simulink model "control_pmsm_multiple"  (R2023a)
settings: Solver=FixedStepAuto  StartTime=0.0  StopTime=0.3  RelTol=1e-3  EnableMultiTasking=on
undefined symbols (not defined in the file): ControlModes, EstimationVelocityModes
settings Model: DataDictionary=EmbeddedBoardDD.sldd  SimulationMode=accelerator  Creator=upattacini  LastModifiedBy=mfussi
settings SolverCC: AllowMultiTaskInputOutput=on  AutoInsertRateTranBlk=on  InsertRTBMode=Never (minimum delay)  EnableFixedStepZeroCrossing=on
settings DataIOCC: SaveOutput=off  DSMLogging=off  SaveTime=off  ReturnWorkspaceOutputs=off
settings OptimizationCC: SimCompilerOptimization=on
settings DebuggingCC: ParameterPrecisionLossMsg=none  UnconnectedInputMsg=warning  UnconnectedOutputMsg=warning  UnconnectedLineMsg=warning
settings ModelReferenceCC: EnableRefExpFcnMdlSchedulingChecks=on
settings RTWCC: DLArmComputeVersion=19.05

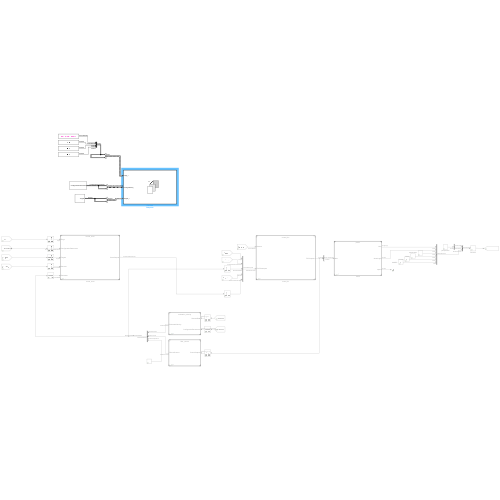
[thumbnail: Simulink's stored preview of the top-level diagram]
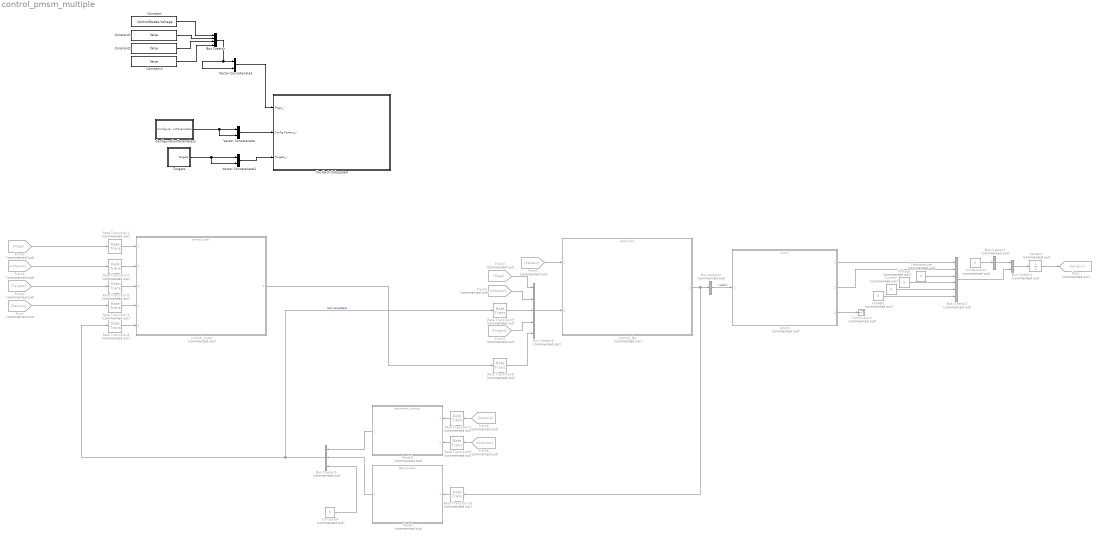
== system control_pmsm_multiple ==
  Bus Creator : BusCreator  Inputs=4  OutDataTypeStr=Bus: Flags  NonVirtualBus=on
      settings: InheritFromInputs=off
  Bus Creator1 : BusCreator  Commented=on  Inputs=2  OutDataTypeStr=Bus: SensorsData  NonVirtualBus=on
      settings: InheritFromInputs=off
  Bus Creator2 : BusCreator  Commented=on  Inputs=6  OutDataTypeStr=Bus: MotorSensors  NonVirtualBus=on
      settings: InheritFromInputs=off
  Bus Creator3 : BusCreator  Commented=on  Inputs=1  OutDataTypeStr=Bus: JointPositions  NonVirtualBus=on
      settings: InheritFromInputs=off
  Bus Creator5 : BusCreator  Commented=on  Inputs=3  OutDataTypeStr=Bus: EstimatedData  NonVirtualBus=on
      settings: InheritFromInputs=off
  Bus Creator6 : BusCreator  Commented=on  Inputs=5  OutDataTypeStr=Bus: FOCSlowInputs  NonVirtualBus=on
      settings: InheritFromInputs=off
  Bus Selector : BusSelector  Commented=on  OutputSignals=Vabc
  ConfigurationParameters : Subsystem
  Constant : Constant  Value=ControlModes.Voltage  OutDataTypeStr=Enum: ControlModes  LockScale=on
  Constant1 : Constant  Value=false  OutDataTypeStr=boolean  LockScale=on
  Constant2 : Constant  Value=false  OutDataTypeStr=boolean  LockScale=on
  Constant3 : Constant  Value=false  OutDataTypeStr=boolean  LockScale=on
  Constant4 : Constant  Commented=on  Value=0  OutDataTypeStr=Bus: MotorTemperature
  Current : Constant  Commented=on  Value=0  OutDataTypeStr=single
  For Each Subsystem : Subsystem  TreatAsAtomicUnit=on
  From : From  Commented=on  GotoTag=Sensors
  From1 : From  Commented=on  GotoTag=Sensors
  From2 : From  Commented=on  GotoTag=Targets
  From3 : From  Commented=on  GotoTag=Targets
  From4 : From  Commented=on  GotoTag=Configuration
  From5 : From  Commented=on  GotoTag=Configuration
  From6 : From  Commented=on  GotoTag=Flags
  From7 : From  Commented=on  GotoTag=Flags
  From8 : From  Commented=on  GotoTag=Configuration
  From9 : From  Commented=on  GotoTag=Sensors
  Goto : Goto  Commented=on  GotoTag=Sensors
  Model : ModelReference  Commented=on  ModelNameDialog=filter_current.slx  SimulationMode=Normal  ModelReferenceVersion=5.1
  Model1 : ModelReference  Commented=on  ModelNameDialog=estimation_velocity.slx  SimulationMode=Normal  ModelReferenceVersion=5.1
  Rate Transition{1..10} (10 alike) : RateTransition  Commented=on  Deterministic=off
  Sensors : UnitDelay  Commented=on  SampleTime=-1  HasFrameUpgradeWarning=on
  Targets : Subsystem
  Temperature : Constant  Commented=on  Value=0  OutDataTypeStr=single
  Terminator1 : Terminator  Commented=on
  Vector Concatenate : Concatenate
  Vector Concatenate1 : Concatenate
  Vector Concatenate2 : Concatenate
  Voltage : Constant  Commented=on  Value=0  OutDataTypeStr=single
  control_foc : ModelReference  Commented=on  ModelNameDialog=control_foc.slx  SimulationMode=Normal  ModelReferenceVersion=5.12
  control_outer : ModelReference  Commented=on  ModelNameDialog=control_outer.slx  SimulationMode=Normal  ModelReferenceVersion=5.5
  hallABC : Constant  Commented=on  Value=0  OutDataTypeStr=uint8
  jointposition : Constant  Commented=on  Value=0  OutDataTypeStr=single
  pmsm : ModelReference  Commented=on  ModelNameDialog=pmsm.slx  SimulationMode=Normal  ModelReferenceVersion=6.0
  wires:
  control_foc/1 -> Rate Transition10/1, Bus Selector/1
  Bus Selector/1 -> pmsm/1  "<Vabc>"
  Constant/1 -> Bus Creator/1
  Bus Creator3/1 -> Bus Creator1/1
  jointposition/1 -> Bus Creator3/1
  pmsm/1 -> Bus Creator2/1
  Temperature/1 -> Bus Creator2/3
  Voltage/1 -> Bus Creator2/4
  Current/1 -> Bus Creator2/5
  hallABC/1 -> Bus Creator2/6
  pmsm/3 -> Terminator1/1
  Bus Creator2/1 -> Bus Creator1/2
  Bus Creator1/1 -> Sensors/1
  ConfigurationParameters/1(ConfigurationParameters) -> Vector Concatenate/2, Vector Concatenate/1
  pmsm/2 -> Bus Creator2/2
  Sensors/1 -> Goto/1
  From6/1 -> Rate Transition1/1
  Rate Transition1/1 -> control_outer/1
  Rate Transition2/1 -> control_outer/2
  From4/1 -> Rate Transition2/1
  Rate Transition3/1 -> control_outer/4
  From/1 -> Rate Transition3/1
  Rate Transition4/1 -> control_outer/5
  Rate Transition5/1 -> control_outer/3
  From2/1 -> Rate Transition5/1
  control_outer/1 -> Rate Transition6/1
  Bus Creator6/1 -> control_foc/2
  From3/1 -> Bus Creator6/4
  Rate Transition6/1 -> Bus Creator6/5
  Bus Creator5/1 -> Rate Transition9/1, Rate Transition4/1  "EstimatedData"
  From5/1 -> Bus Creator6/2
  From7/1 -> Bus Creator6/1
  From1/1 -> control_foc/1
  Constant1/1 -> Bus Creator/2
  Constant2/1 -> Bus Creator/3
  Model1/1 -> Bus Creator5/1
  Model/1 -> Bus Creator5/2
  From8/1 -> Rate Transition8/1
  From9/1 -> Rate Transition7/1
  Rate Transition7/1 -> Model1/1
  Rate Transition8/1 -> Model1/2
  Rate Transition9/1 -> Bus Creator6/3
  Rate Transition10/1 -> Model/1
  Constant3/1 -> Bus Creator/4
  Constant4/1 -> Bus Creator5/3
  Vector Concatenate/1 -> For Each Subsystem/2(Config Params_i)
  Bus Creator/1 -> Vector Concatenate1/2, Vector Concatenate1/1
  Vector Concatenate1/1 -> For Each Subsystem/1(Flags_i)
  Vector Concatenate2/1 -> For Each Subsystem/3(Targets_i)
  Targets/1(Targets) -> Vector Concatenate2/2, Vector Concatenate2/1

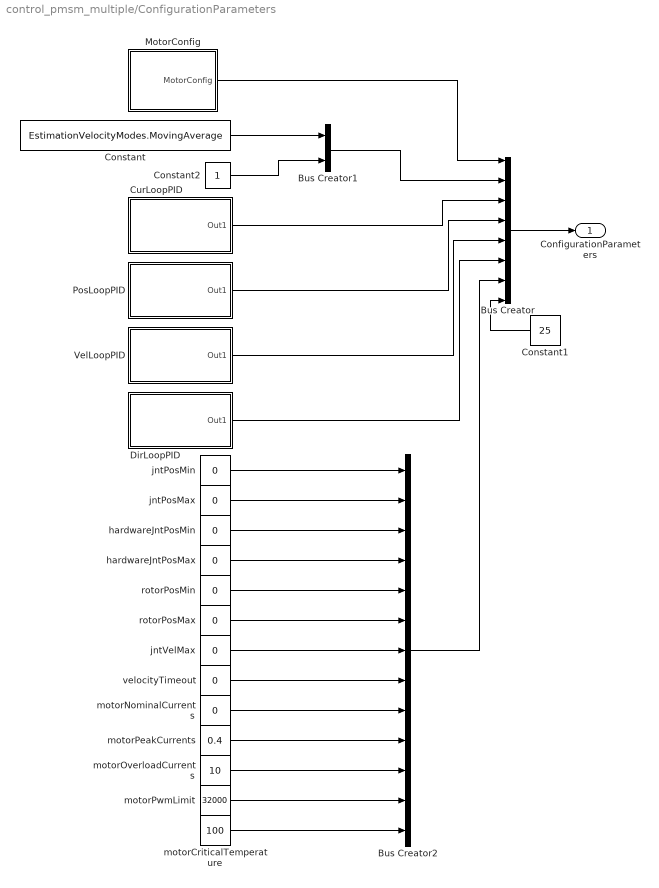
== system control_pmsm_multiple/ConfigurationParameters ==
  Bus Creator : BusCreator  Inputs=8  OutDataTypeStr=Bus: ConfigurationParameters  NonVirtualBus=on
      settings: InheritFromInputs=off
  Bus Creator1 : BusCreator  Inputs=2  OutDataTypeStr=Bus: EstimationConfig  NonVirtualBus=on
      settings: InheritFromInputs=off
  Bus Creator2 : BusCreator  Inputs=13  OutDataTypeStr=Bus: Thresholds  NonVirtualBus=on
      settings: InheritFromInputs=off
  Constant : Constant  Value=EstimationVelocityModes.MovingAverage  OutDataTypeStr=Enum: EstimationVelocityModes
  Constant1 : Constant  Value=25  OutDataTypeStr=single
  Constant2 : Constant  OutDataTypeStr=single
  CurLoopPID : Subsystem  mask{OutMax=0, OutMin=0, P=2, I=500, D=0, N=10, I0=0, D0=0, shift_factor=0}
      mask prompts: shift_factor "Shift Factor"
  DirLoopPID : Subsystem  mask{OutMax=0, OutMin=0, P=0, I=0, D=0, N=0, I0=0, D0=0, shift_factor=0}
      mask prompts: shift_factor "Shift Factor"
  MotorConfig : Subsystem  mask{has_hall_sens=true, has_quadrature_encoder=true, has_speed_quadrature_encoder=false, has_torque_sens=false, use_index=true, enable_verbosity=false, rotor_encoder_resolution=16000, rotor_index_offset=0, encoder_tolerance=0, pole_pairs=7, reduction=1, Kbemf=0, Rphase=0, Imin=-10, Imax=10, Vcc=24, Vmax=24, R=29.5, L=200, Rt=50, tau=200}
      mask prompts: R "Motor Resistance"; L "Motor Inductance"; Rt "Thermal Resistance"; tau "Thermal Time Constant"
  PosLoopPID : Subsystem  mask{OutMax=0, OutMin=0, P=0, I=0, D=0, N=0, I0=0, D0=0, shift_factor=0}
      mask prompts: shift_factor "Shift Factor"
  VelLoopPID : Subsystem  mask{OutMax=0, OutMin=0, P=0, I=0, D=0, N=0, I0=0, D0=0, shift_factor=0}
      mask prompts: shift_factor "Shift Factor"
  hardwareJntPosMax : Constant  Value=0  OutDataTypeStr=single
  hardwareJntPosMin : Constant  Value=0  OutDataTypeStr=single
  jntPosMax : Constant  Value=0  OutDataTypeStr=single
  jntPosMin : Constant  Value=0  OutDataTypeStr=single
  jntVelMax : Constant  Value=0  OutDataTypeStr=single
  motorCriticalTemperature : Constant  Value=100  OutDataTypeStr=single
  motorNominalCurrents : Constant  Value=0  OutDataTypeStr=single
  motorOverloadCurrents : Constant  Value=10  OutDataTypeStr=single
  motorPeakCurrents : Constant  Value=0.4  OutDataTypeStr=single
  motorPwmLimit : Constant  Value=32000  OutDataTypeStr=uint32
  rotorPosMax : Constant  Value=0  OutDataTypeStr=single
  rotorPosMin : Constant  Value=0  OutDataTypeStr=single
  velocityTimeout : Constant  Value=0  OutDataTypeStr=uint32
  ConfigurationParameters : Outport
  wires:
  Bus Creator/1 -> ConfigurationParameters/1
  Constant/1 -> Bus Creator1/1
  jntPosMin/1 -> Bus Creator2/1
  jntPosMax/1 -> Bus Creator2/2
  hardwareJntPosMin/1 -> Bus Creator2/3
  hardwareJntPosMax/1 -> Bus Creator2/4
  rotorPosMin/1 -> Bus Creator2/5
  rotorPosMax/1 -> Bus Creator2/6
  jntVelMax/1 -> Bus Creator2/7
  velocityTimeout/1 -> Bus Creator2/8
  motorNominalCurrents/1 -> Bus Creator2/9
  motorPeakCurrents/1 -> Bus Creator2/10
  motorOverloadCurrents/1 -> Bus Creator2/11
  motorPwmLimit/1 -> Bus Creator2/12
  Bus Creator1/1 -> Bus Creator/2
  PosLoopPID/1(Out1) -> Bus Creator/4
  CurLoopPID/1(Out1) -> Bus Creator/3
  VelLoopPID/1(Out1) -> Bus Creator/5
  MotorConfig/1(MotorConfig) -> Bus Creator/1
  DirLoopPID/1(Out1) -> Bus Creator/6
  Bus Creator2/1 -> Bus Creator/7
  Constant1/1 -> Bus Creator/8
  motorCriticalTemperature/1 -> Bus Creator2/13
  Constant2/1 -> Bus Creator1/2

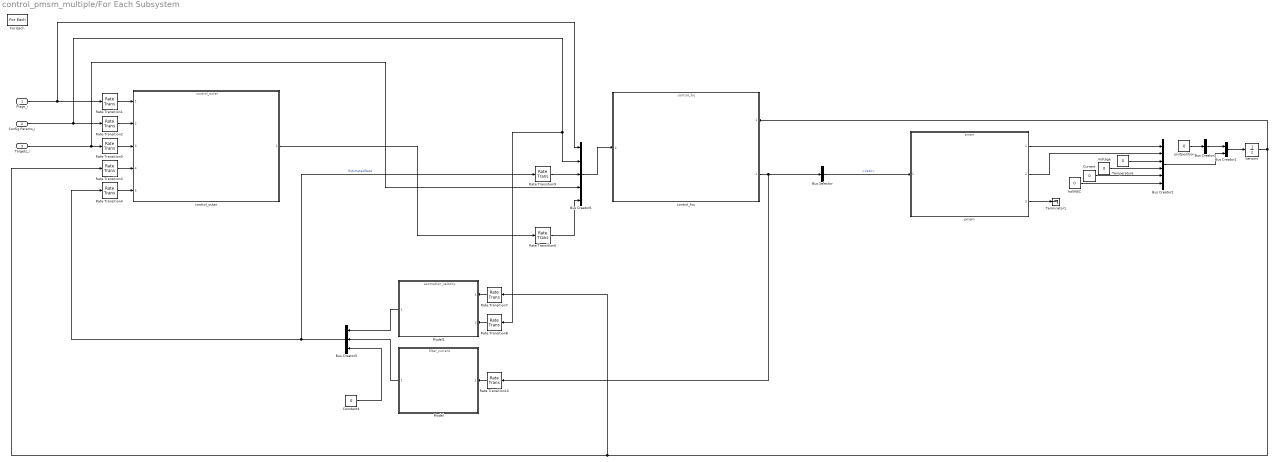
== system control_pmsm_multiple/For Each Subsystem ==
  Flags_i : Inport  OutDataTypeStr=Bus: Flags  Partition=on  PartitionDimension=1  PartitionWidth=1  PartitionOffset=0
  Config Params_i : Inport  Port=2  Partition=on  PartitionDimension=1  PartitionWidth=1  PartitionOffset=0
  Targets_i : Inport  Port=3  Partition=on  PartitionDimension=1  PartitionWidth=1  PartitionOffset=0
  Bus Creator1 : BusCreator  Inputs=2  OutDataTypeStr=Bus: SensorsData  NonVirtualBus=on
      settings: InheritFromInputs=off
  Bus Creator2 : BusCreator  Inputs=6  OutDataTypeStr=Bus: MotorSensors  NonVirtualBus=on
      settings: InheritFromInputs=off
  Bus Creator3 : BusCreator  Inputs=1  OutDataTypeStr=Bus: JointPositions  NonVirtualBus=on
      settings: InheritFromInputs=off
  Bus Creator5 : BusCreator  Inputs=3  OutDataTypeStr=Bus: EstimatedData  NonVirtualBus=on
      settings: InheritFromInputs=off
  Bus Creator6 : BusCreator  Inputs=5  OutDataTypeStr=Bus: FOCSlowInputs  NonVirtualBus=on
      settings: InheritFromInputs=off
  Bus Selector : BusSelector  OutputSignals=Vabc
  Constant4 : Constant  Value=0  OutDataTypeStr=Bus: MotorTemperature
  Current : Constant  Value=0  OutDataTypeStr=single
  For Each : ForEach  DisableCoverage=on
  Model : ModelReference  ModelNameDialog=filter_current.slx  ModelReferenceVersion=5.1
  Model1 : ModelReference  ModelNameDialog=estimation_velocity.slx  ModelReferenceVersion=5.1
  Rate Transition{1..10} (10 alike) : RateTransition  Deterministic=off
  Sensors : UnitDelay  SampleTime=-1  HasFrameUpgradeWarning=on
  Temperature : Constant  Value=0  OutDataTypeStr=single
  Terminator1 : Terminator
  Voltage : Constant  Value=0  OutDataTypeStr=single
  control_foc : ModelReference  ModelNameDialog=control_foc.slx  ModelReferenceVersion=5.12
      settings: PortSchema="{\"entries\":[{\"content\":{\"sides\":[{\"content\":{\"connectorIds\":[\"In2\"]},\"type\":\"ConnectorPlacement.EquallySpacedRectSide\",\"uuid\":\"ad3e0007-7e1a-45e3-9c4b-8557c15e59c9\"},{\"content\":{\"connectorIds\":[\"In1\",\"Out1\"],\"side\":\"RIGHT\"},\"type\":\"ConnectorPlacement.EquallySpacedRectSide\",\"uuid\":\"9939f2ed-714d-478a-b916-4c98246d3dad\"},{\"content\":{\"side\":\"TOP\"},\"type\":\"ConnectorPlacement.EquallySpacedRectSide\",\"uuid\":\"1f2bf02e-7550-4331-be09-78a4da3cd08c\"}]},\"type\":\"ConnectorPlacement.EquallySpacedConnector\",\"uuid\":\"c84d0359-7250-4a6f-b291-6b1b96be2690\"}],\"packageUris\":[\"http://schema.mathworks.com/mf0/Connector/R2020b\"],\"version\":\"1.0\"}"
  control_outer : ModelReference  ModelNameDialog=control_outer.slx  ModelReferenceVersion=5.5
  hallABC : Constant  Value=0  OutDataTypeStr=uint8
  jointposition : Constant  Value=0  OutDataTypeStr=single
  pmsm : ModelReference  ModelNameDialog=pmsm.slx  ModelReferenceVersion=6.0
  wires:
  Rate Transition8/1 -> Model1/2
  Flags_i/1 -> Rate Transition1/1, Bus Creator6/1
  Constant4/1 -> Bus Creator5/3
  Rate Transition9/1 -> Bus Creator6/3
  Bus Creator6/1 -> control_foc/2
  Rate Transition2/1 -> control_outer/2
  Sensors/1 -> Rate Transition7/1, Rate Transition3/1, control_foc/1
  Config Params_i/1 -> Rate Transition2/1, Bus Creator6/2, Rate Transition8/1
  Targets_i/1 -> Bus Creator6/4, Rate Transition5/1
  Rate Transition4/1 -> control_outer/5
  Model/1 -> Bus Creator5/2
  control_outer/1 -> Rate Transition6/1
  Rate Transition6/1 -> Bus Creator6/5
  Rate Transition7/1 -> Model1/1
  Bus Creator5/1 -> Rate Transition9/1, Rate Transition4/1  "EstimatedData"
  Rate Transition5/1 -> control_outer/3
  Rate Transition1/1 -> control_outer/1
  Rate Transition10/1 -> Model/1
  Rate Transition3/1 -> control_outer/4
  Model1/1 -> Bus Creator5/1
  control_foc/1 -> Bus Selector/1, Rate Transition10/1
  Bus Selector/1 -> pmsm/1  "<Vabc>"
  pmsm/2 -> Bus Creator2/2
  Bus Creator2/1 -> Bus Creator1/2
  Current/1 -> Bus Creator2/5
  Temperature/1 -> Bus Creator2/3
  Voltage/1 -> Bus Creator2/4
  pmsm/1 -> Bus Creator2/1
  jointposition/1 -> Bus Creator3/1
  Bus Creator3/1 -> Bus Creator1/1
  pmsm/3 -> Terminator1/1
  Bus Creator1/1 -> Sensors/1
  hallABC/1 -> Bus Creator2/6

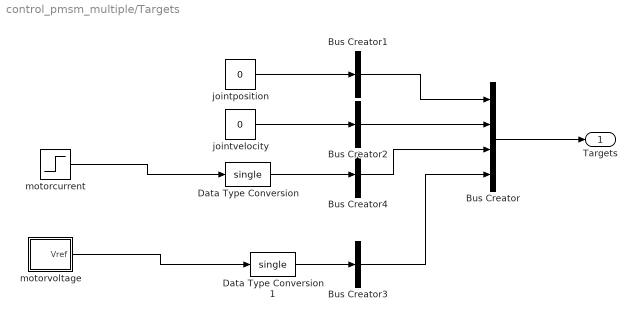
== system control_pmsm_multiple/Targets ==
  Bus Creator : BusCreator  Inputs=4  OutDataTypeStr=Bus: Targets  NonVirtualBus=on
      settings: InheritFromInputs=off
  Bus Creator1 : BusCreator  Inputs=1  OutDataTypeStr=Bus: JointPositions  NonVirtualBus=on
      settings: InheritFromInputs=off
  Bus Creator2 : BusCreator  Inputs=1  OutDataTypeStr=Bus: JointVelocities  NonVirtualBus=on
      settings: InheritFromInputs=off
  Bus Creator3 : BusCreator  Inputs=1  OutDataTypeStr=Bus: MotorVoltage  NonVirtualBus=on
      settings: InheritFromInputs=off
  Bus Creator4 : BusCreator  Inputs=1  OutDataTypeStr=Bus: MotorCurrent  NonVirtualBus=on
      settings: InheritFromInputs=off
  Data Type Conversion : DataTypeConversion  OutDataTypeStr=single  SaturateOnIntegerOverflow=off  RndMeth=Floor
  Data Type Conversion1 : DataTypeConversion  OutDataTypeStr=single  SaturateOnIntegerOverflow=off  RndMeth=Floor
  jointposition : Constant  Value=0  OutDataTypeStr=single
  jointvelocity : Constant  Value=0  OutDataTypeStr=single
  motorcurrent : Step  Time=0.1  After=0.8  SampleTime=0
  motorvoltage : Subsystem
  Targets : Outport
  wires:
  Bus Creator/1 -> Targets/1
  jointposition/1 -> Bus Creator1/1
  Bus Creator1/1 -> Bus Creator/1
  Bus Creator2/1 -> Bus Creator/2
  Bus Creator3/1 -> Bus Creator/4
  Bus Creator4/1 -> Bus Creator/3
  jointvelocity/1 -> Bus Creator2/1
  Data Type Conversion1/1 -> Bus Creator3/1
  Data Type Conversion/1 -> Bus Creator4/1
  motorcurrent/1 -> Data Type Conversion/1
  motorvoltage/1(Vref) -> Data Type Conversion1/1

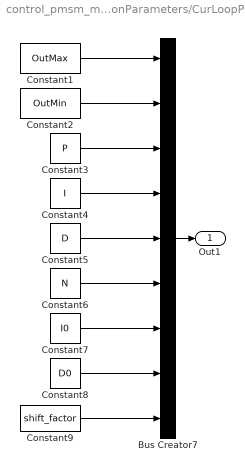
== system control_pmsm_multiple/ConfigurationParameters/CurLoopPID ==
  Bus Creator7 : BusCreator  Inputs=9  OutDataTypeStr=Bus: PIDConfig  NonVirtualBus=on
      settings: InheritFromInputs=off
  Constant1 : Constant  Value=OutMax  OutDataTypeStr=single
  Constant2 : Constant  Value=OutMin  OutDataTypeStr=single
  Constant3 : Constant  Value=P  OutDataTypeStr=single
  Constant4 : Constant  Value=I  OutDataTypeStr=single
  Constant5 : Constant  Value=D  OutDataTypeStr=single
  Constant6 : Constant  Value=N  OutDataTypeStr=single
  Constant7 : Constant  Value=I0  OutDataTypeStr=single
  Constant8 : Constant  Value=D0  OutDataTypeStr=single
  Constant9 : Constant  Value=shift_factor  OutDataTypeStr=uint8
  Out1 : Outport
  wires:
  Constant9/1 -> Bus Creator7/9
  Constant5/1 -> Bus Creator7/5
  Bus Creator7/1 -> Out1/1
  Constant8/1 -> Bus Creator7/8
  Constant2/1 -> Bus Creator7/2
  Constant4/1 -> Bus Creator7/4
  Constant7/1 -> Bus Creator7/7
  Constant1/1 -> Bus Creator7/1
  Constant3/1 -> Bus Creator7/3
  Constant6/1 -> Bus Creator7/6

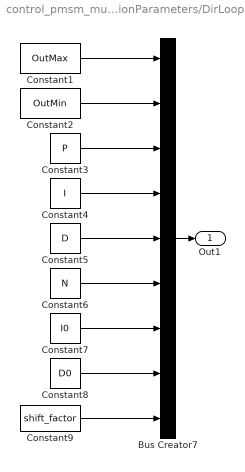
== system control_pmsm_multiple/ConfigurationParameters/DirLoopPID ==
  Bus Creator7 : BusCreator  Inputs=9  OutDataTypeStr=Bus: PIDConfig  NonVirtualBus=on
      settings: InheritFromInputs=off
  Constant1 : Constant  Value=OutMax  OutDataTypeStr=single
  Constant2 : Constant  Value=OutMin  OutDataTypeStr=single
  Constant3 : Constant  Value=P  OutDataTypeStr=single
  Constant4 : Constant  Value=I  OutDataTypeStr=single
  Constant5 : Constant  Value=D  OutDataTypeStr=single
  Constant6 : Constant  Value=N  OutDataTypeStr=single
  Constant7 : Constant  Value=I0  OutDataTypeStr=single
  Constant8 : Constant  Value=D0  OutDataTypeStr=single
  Constant9 : Constant  Value=shift_factor  OutDataTypeStr=uint8
  Out1 : Outport
  wires:
  Constant6/1 -> Bus Creator7/6
  Constant3/1 -> Bus Creator7/3
  Constant1/1 -> Bus Creator7/1
  Constant7/1 -> Bus Creator7/7
  Constant4/1 -> Bus Creator7/4
  Constant2/1 -> Bus Creator7/2
  Constant8/1 -> Bus Creator7/8
  Bus Creator7/1 -> Out1/1
  Constant5/1 -> Bus Creator7/5
  Constant9/1 -> Bus Creator7/9

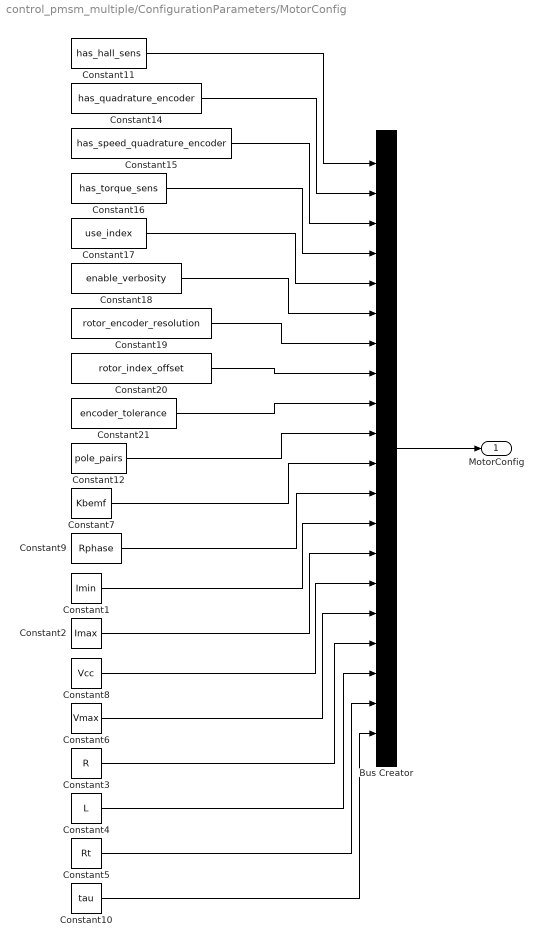
== system control_pmsm_multiple/ConfigurationParameters/MotorConfig ==
  Bus Creator : BusCreator  Inputs=20  OutDataTypeStr=Bus: MotorConfig  NonVirtualBus=on
      settings: InheritFromInputs=off
  Constant1 : Constant  Value=Imin  OutDataTypeStr=single
  Constant10 : Constant  Value=tau  OutDataTypeStr=single
  Constant11 : Constant  Value=has_hall_sens  OutDataTypeStr=boolean
  Constant12 : Constant  Value=pole_pairs  OutDataTypeStr=uint8
  Constant14 : Constant  Value=has_quadrature_encoder  OutDataTypeStr=boolean
  Constant15 : Constant  Value=has_speed_quadrature_encoder  OutDataTypeStr=boolean
  Constant16 : Constant  Value=has_torque_sens  OutDataTypeStr=boolean
  Constant17 : Constant  Value=use_index  OutDataTypeStr=boolean
  Constant18 : Constant  Value=enable_verbosity  OutDataTypeStr=boolean
  Constant19 : Constant  Value=rotor_encoder_resolution  OutDataTypeStr=int16
  Constant2 : Constant  Value=Imax  OutDataTypeStr=single
  Constant20 : Constant  Value=rotor_index_offset  OutDataTypeStr=int16
  Constant21 : Constant  Value=encoder_tolerance  OutDataTypeStr=uint8
  Constant3 : Constant  Value=R  OutDataTypeStr=single
  Constant4 : Constant  Value=L  OutDataTypeStr=single
  Constant5 : Constant  Value=Rt  OutDataTypeStr=single
  Constant6 : Constant  Value=Vmax  OutDataTypeStr=single
  Constant7 : Constant  Value=Kbemf  OutDataTypeStr=single
  Constant8 : Constant  Value=Vcc  OutDataTypeStr=single
  Constant9 : Constant  Value=Rphase  OutDataTypeStr=single
  MotorConfig : Outport
  wires:
  Bus Creator/1 -> MotorConfig/1
  Constant20/1 -> Bus Creator/8
  Constant19/1 -> Bus Creator/7
  Constant21/1 -> Bus Creator/9
  Constant15/1 -> Bus Creator/3
  Constant18/1 -> Bus Creator/6
  Constant14/1 -> Bus Creator/2
  Constant16/1 -> Bus Creator/4
  Constant17/1 -> Bus Creator/5
  Constant12/1 -> Bus Creator/10
  Constant11/1 -> Bus Creator/1
  Constant7/1 -> Bus Creator/11
  Constant9/1 -> Bus Creator/12
  Constant1/1 -> Bus Creator/13
  Constant2/1 -> Bus Creator/14
  Constant8/1 -> Bus Creator/15
  Constant6/1 -> Bus Creator/16
  Constant3/1 -> Bus Creator/17
  Constant4/1 -> Bus Creator/18
  Constant5/1 -> Bus Creator/19
  Constant10/1 -> Bus Creator/20

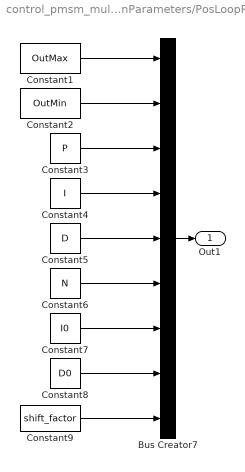
== system control_pmsm_multiple/ConfigurationParameters/PosLoopPID ==
  Bus Creator7 : BusCreator  Inputs=9  OutDataTypeStr=Bus: PIDConfig  NonVirtualBus=on
      settings: InheritFromInputs=off
  Constant1 : Constant  Value=OutMax  OutDataTypeStr=single
  Constant2 : Constant  Value=OutMin  OutDataTypeStr=single
  Constant3 : Constant  Value=P  OutDataTypeStr=single
  Constant4 : Constant  Value=I  OutDataTypeStr=single
  Constant5 : Constant  Value=D  OutDataTypeStr=single
  Constant6 : Constant  Value=N  OutDataTypeStr=single
  Constant7 : Constant  Value=I0  OutDataTypeStr=single
  Constant8 : Constant  Value=D0  OutDataTypeStr=single
  Constant9 : Constant  Value=shift_factor  OutDataTypeStr=uint8
  Out1 : Outport
  wires:
  Constant6/1 -> Bus Creator7/6
  Constant3/1 -> Bus Creator7/3
  Constant1/1 -> Bus Creator7/1
  Constant7/1 -> Bus Creator7/7
  Constant4/1 -> Bus Creator7/4
  Constant2/1 -> Bus Creator7/2
  Constant8/1 -> Bus Creator7/8
  Bus Creator7/1 -> Out1/1
  Constant5/1 -> Bus Creator7/5
  Constant9/1 -> Bus Creator7/9

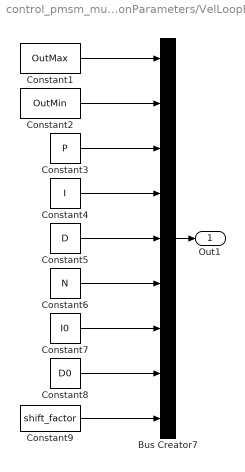
== system control_pmsm_multiple/ConfigurationParameters/VelLoopPID ==
  Bus Creator7 : BusCreator  Inputs=9  OutDataTypeStr=Bus: PIDConfig  NonVirtualBus=on
      settings: InheritFromInputs=off
  Constant1 : Constant  Value=OutMax  OutDataTypeStr=single
  Constant2 : Constant  Value=OutMin  OutDataTypeStr=single
  Constant3 : Constant  Value=P  OutDataTypeStr=single
  Constant4 : Constant  Value=I  OutDataTypeStr=single
  Constant5 : Constant  Value=D  OutDataTypeStr=single
  Constant6 : Constant  Value=N  OutDataTypeStr=single
  Constant7 : Constant  Value=I0  OutDataTypeStr=single
  Constant8 : Constant  Value=D0  OutDataTypeStr=single
  Constant9 : Constant  Value=shift_factor  OutDataTypeStr=uint8
  Out1 : Outport
  wires:
  Constant9/1 -> Bus Creator7/9
  Constant5/1 -> Bus Creator7/5
  Bus Creator7/1 -> Out1/1
  Constant8/1 -> Bus Creator7/8
  Constant2/1 -> Bus Creator7/2
  Constant4/1 -> Bus Creator7/4
  Constant7/1 -> Bus Creator7/7
  Constant1/1 -> Bus Creator7/1
  Constant3/1 -> Bus Creator7/3
  Constant6/1 -> Bus Creator7/6

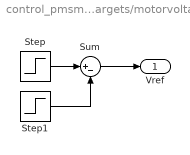
== system control_pmsm_multiple/Targets/motorvoltage ==
  Step : Step  Time=0.1  After=30  SampleTime=0
  Step1 : Step  Time=0.2  After=15  SampleTime=0
  Sum : Sum  Inputs=|+-
  Vref : Outport
  wires:
  Sum/1 -> Vref/1
  Step1/1 -> Sum/2
  Step/1 -> Sum/1
